simulink model "DCM_16_Series_Field_2"  (R2019b)
settings: Solver=VariableStepAuto  StartTime=0.0  StopTime=20  RelTol=1e-3
model workspace (MAT data in the model file):
  Laf = 0.00847
  Rarm = 0.0096
  angular_vel = 165
  angular_vel_13 = 163.55
  angular_vel_14 = 163.55
  angular_vel_15 = 163.55
  angular_vel_16 = 163.55
  angular_vel_2 = 165
libraries: powerlib x77, simulink x1
settings Model: Creator=Sy2  LastModifiedBy=Sy2
settings SolverCC: ZeroCrossAlgorithm=Adaptive
settings DebuggingCC: IgnoredZcDiagnostic=none

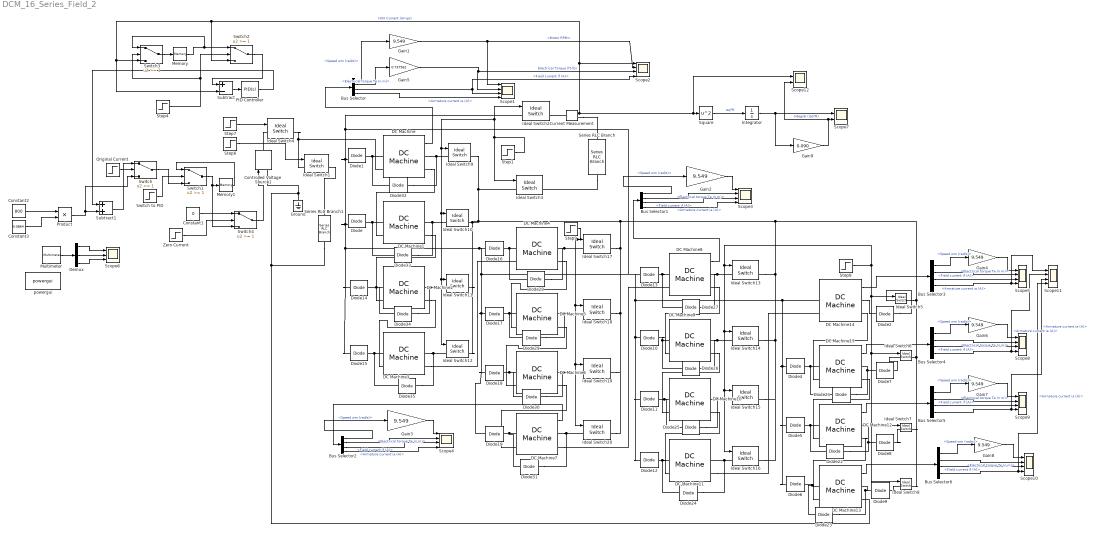
== system DCM_16_Series_Field_2 ==
  Bus Selector{,1..6} (7 alike) : BusSelector  OutputSignals=Speed wm (rad/s),Electrical torque Te (n m),Field current if (A),Armature current ia (A)
  Constant1 : Constant  Value=0
  Constant2 : Constant  Value=800
  Constant3 : Constant  Value=0.0864
  Controlled Voltage Source1 : powerlib/Electrical Sources/Controlled Voltage Source  Initialize=on  Source_Type=DC  Amplitude=0  Phase=0  Frequency=0  Measurements=Voltage
      settings: SourceProductName=Simscape Electrical
  Current Measurement : powerlib/Measurements/Current Measurement  PhasorSimulation=off  OutputType=Complex  PSBequivalent=0
      settings: SourceProductName=Simscape Electrical
  DC Machine{,1..13,15} (15 alike) : powerlib/Machines/DC Machine  PresetModel=No  MechanicalLoad=Torque TL  FieldType=Wound  ShowDetailedParameters=on  MeasurementBus=off  RLa="[Rarm  0.002]"  RLf=[0.0054 0.0125]  Laf=Laf  MachineConstant=Torque constant (N.m/A)  Ke=1.8  Kt=1.8  J=137  Bm=0  Tf=0  w0=angular_vel  Ifinit=0  TsPowergui=0  TsBlock=-1
      settings: SourceProductName=Simscape Electrical
  DC Machine14 : powerlib/Machines/DC Machine  PresetModel=No  MechanicalLoad=Torque TL  FieldType=Wound  ShowDetailedParameters=on  MeasurementBus=off  RLa="[Rarm  0.002]"  RLf=[0.0054 0.0125]  Laf=Laf  MachineConstant=Torque constant (N.m/A)  Ke=1.8  Kt=1.8  J=137  Bm=0  Tf=0  w0=angular_vel_13  Ifinit=0  TsPowergui=0  TsBlock=-1
      settings: SourceProductName=Simscape Electrical
  Demux : Demux  Outputs=3
  Diode : powerlib/Power Electronics/Diode  Ron=0.001  Lon=0  Vf=0.8  IC=0  UseSnubber=0  Rs=500  Cs=250e-9  Measurements=on
      settings: SourceProductName=Simscape Electrical
  Diode1 : powerlib/Power Electronics/Diode  Ron=0.001  Lon=0  Vf=0.8  IC=0  UseSnubber=0  Rs=500  Cs=250e-9  Measurements=on
      settings: SourceProductName=Simscape Electrical
  Diode{2,4..19,21..22} (19 alike) : powerlib/Power Electronics/Diode  Ron=0.001  Lon=0  Vf=0.8  IC=0  UseSnubber=0  Rs=500  Cs=250e-9  Measurements=off
      settings: SourceProductName=Simscape Electrical
  Diode{23..35} (13 alike) : powerlib/Power Electronics/Diode  Ron=0  Lon=0  Vf=0.8  IC=0  UseSnubber=0  Rs=500  Cs=250e-9  Measurements=off
      settings: SourceProductName=Simscape Electrical
  Gain{1..4,6..8} (7 alike) : Gain  Gain=9.549
  Gain5 : Gain  Gain=0.737562
  Gain9 : Gain  Gain=0.090
  Ground : powerlib/Elements/Ground  LConnTagsString=a
      settings: SourceProductName=Simscape Electrical
  Ideal Switch{1..3,5..20} (19 alike) : powerlib/Power Electronics/Ideal Switch  Ron=0  Lon=0  IC=0  Rs=inf  Cs=0  Measurements=on
      settings: SourceProductName=Simscape Electrical
  Ideal Switch4 : powerlib/Power Electronics/Ideal Switch  Ron=0  Lon=0  IC=1  Rs=inf  Cs=0  Measurements=on
      settings: SourceProductName=Simscape Electrical
  Integrator : Integrator  ZeroCross=off
  Memory : Memory
  Memory1 : Memory
  Multimeter : powerlib/Measurements/Multimeter  PhasorSimulation=off  OutputType=Complex  sel=[2 3 1]  L=3  Gain=[1 1 1]  yselected={'Usrc: Controlled Voltage Source1','Ib: Series RLC Branch1','Ub: Series RLC Branch1'};  PSBOutputType=1  PSBequivalent=0  AxesSetting=[0,0.1,-100,100]  Display=0  SavedBlockNames=-11
      settings: SourceProductName=Simscape Electrical
  Original Current : Step  Time=13  SampleTime=0  VectorParams1D=off  ZeroCross=off
  PID Controller : simulink/Continuous/PID Controller  Controller=PID  Form=Parallel  TimeDomain=Continuous-time  SampleTime=-1  IntegratorMethod=Forward Euler  FilterMethod=Forward Euler  ControllerParametersSource=internal  P=10  I=7  D=1  UseFilter=on  N=100  TunerSelectOption=Transfer Function Based (PID Tuner App)  InitialConditionSource=internal  InitialConditionForIntegrator=0  InitialConditionForFilter=0  DifferentiatorICPrevScaledInput=0  ExternalReset=none  TrackingMode=off  Kt=1  LimitOutput=off  UpperSaturationLimit=inf  LowerSaturationLimit=-inf  LinearizeAsGain=on  AntiWindupMode=none  Kb=1  POutMin=[]  POutMax=[]  IOutMin=[]  IOutMax=[]  DOutMin=[]  DOutMax=[]  NOutMin=[]  NOutMax=[]  SumOutMin=[]  SumOutMax=[]  SaturationOutMin=[]  SaturationOutMax=[]  PParamMin=[]  PParamMax=[]  IParamMin=[]  IParamMax=[]  DParamMin=[]  DParamMax=[]  NParamMin=[]  NParamMax=[]  KbParamMin=[]  KbParamMax=[]  KtParamMin=[]  KtParamMax=[]  KbOutMin=[]  KbOutMax=[]  KtOutMin=[]  KtOutMax=[]  IntegratorOutMin=[]  IntegratorOutMax=[]  FilterOutMin=[]  FilterOutMax=[]  SumI1OutMin=[]  SumI1OutMax=[]  SumI2OutMin=[]  SumI2OutMax=[]  SumI3OutMin=[]  SumI3OutMax=[]  SumI4OutMin=[]  SumI4OutMax=[]  SumDOutMin=[]  SumDOutMax=[]  DifferentiatorOutMin=[]  DifferentiatorOutMax=[]  FilterDiffOutCoefMin=[]  FilterDiffOutCoefMax=[]  ReciprocalOutMin=[]  ReciprocalOutMax=[]  SumDenOutMin=[]  SumDenOutMax=[]  SumNumOutMin=[]  SumNumOutMax=[]  DivideOutMin=[]  DivideOutMax=[]  IntegratorContinuousStateAttributes=''  IntegratorStateMustResolveToSignalObject=off  IntegratorRTWStateStorageClass=Auto  FilterContinuousStateAttributes=''  FilterStateMustResolveToSignalObject=off  FilterRTWStateStorageClass=Auto  ParallelPVariant=InternalParameters  IdealPVariant=Disabled  IVariant=InternalParameters  DVariant=InternalParameters  IntegratorVariant=Continuous  SatVariant=Disabled  AWVariant=Passthrough  PCopyVariant=Disabled  TRVariant=Disabled  FdbkBlocksVariant=Forward  IdealPFdbkVariant=Disabled  SatFdbkVariant=Disabled  DerivativeFilterVariant=ContFilter  NVariant=InternalParameters  NCopyVariant=Disabled  FilterICVariant=InternalICsFilter  IntegratorICVariant=InternalICs  ExternalResetVariant=Disabled  TRSumVariant=Passthrough  SumFdbkVariant=Disabled  SumVariant=Sum_PID
  Product : Product
  Scope{1..5,8..11} (9 alike) : Scope  NumInputPorts=4
  Scope12 : Scope  NumInputPorts=2
  Scope6 : Scope  NumInputPorts=3
  Scope7 : Scope  NumInputPorts=2
  Series RLC Branch : powerlib/Elements/Series RLC Branch  LConnTagsString=__new0  RConnTagsString=__new0  BranchType=RL  Resistance=0.09  Inductance=0.02  SetiL0=off  InitialCurrent=0  Capacitance=1e-6  Setx0=off  InitialVoltage=0  Measurements=None
      settings: SourceProductName=Simscape Electrical
  Series RLC Branch1 : powerlib/Elements/Series RLC Branch  Description=Field Dump Resistor  LConnTagsString=__new0  RConnTagsString=__new0  BranchType=R  Resistance=5  Inductance=1e-3  SetiL0=off  InitialCurrent=0  Capacitance=1e-6  Setx0=off  InitialVoltage=0  Measurements=Branch voltage and current
      settings: AttributesFormatString=%<Description>  SourceProductName=Simscape Electrical
  Square : Math  Operator=square  RndMeth=Zero  SaturateOnIntegerOverflow=on
  Step1 : Step  Time=12  SampleTime=0  VectorParams1D=off
  Step4 : Step  Time=12.72  SampleTime=0  VectorParams1D=off  ZeroCross=off
  Step6 : Step  Time=12.85  SampleTime=0  VectorParams1D=off  ZeroCross=off
  Step7 : Step  Time=13  Before=1  After=0  SampleTime=0  VectorParams1D=off  ZeroCross=off
  Step8 : Step  Time=12  SampleTime=0  VectorParams1D=off
  Step9 : Step  Time=12  SampleTime=0  VectorParams1D=off
  Subtract : Sum  Inputs=+-
  Subtract1 : Sum
  Switch{,1..4} (5 alike) : Switch  Threshold=1  ZeroCross=off
  Switch to PID : Step  Time=13  SampleTime=0  VectorParams1D=off  ZeroCross=off
  Zero Current : Step  Time=13  SampleTime=0  VectorParams1D=off  ZeroCross=off
  powergui : powerlib/powergui  Priority=1  SimulationMode=Continuous  SampleTime=50e-6  frequency=60  Iterations=50  frequencyindice=0  Pbase=100e6  ErrMax=1e-4  UnitsV=kV  UnitsW=MW  buscounter=0  FunctionMessages=off  echomessages=off  EnableUseOfTLC=off  CurrentSourceSwitches=off  DisableSnubberDevices=off  DisableRonSwitches=off  DisableVfSwitches=off  DisplayEquations=off  AutomaticDiscreteSolvers=off  SolverType=Tustin/Backward Euler (TBE)  Interpol=off  ExternalGateDelay=off  methode=off  Ts=100  x0status=blocks  SPID=on  SwTol=0  HookPort=off  NonlinearTolerance=1e-4  nMaxIteration=100  ContinueOnMaxIteration=off  RestoreLinks=warning  ResistiveCurrentMeasurement=off  Frange=[0:2:500]  Ylog=off  Xlog=on  ShowGrid=off  save=off  variable=ZData  structure=0  ZoomFFT=off  StartTime=0.0  cycles=1  DisplayStyle=1  fundamental=60  FreqAxis=off  MaxFrequency=1000  frequencyindicesteady=1  RmsSteady=1  display=off
      settings: SourceProductName=Simscape Electrical
  wires:
  DC Machine/1 -> Bus Selector/1
  Bus Selector/1 -> Gain1/1  "<Speed wm (rad/s)>"
  Bus Selector/3 -> Scope2/4, Scope1/3  "<Field current if (A)>"
  Bus Selector/4 -> Scope1/4  "<Armature current ia (A)>"
  Gain1/1 -> Scope1/1, Scope2/2  "<Motor RPM>"
  Step1/1 -> Ideal Switch10/1, Ideal Switch11/1, Ideal Switch12/1, Ideal Switch9/1, Ideal Switch2/1, Ideal Switch3/1
  Original Current/1 -> Switch/2
  Current Measurement/1 -> Scope12/1, Square/1, Switch2/3, Switch3/3, Subtract/2, Scope2/1  "HSX Current (Amps)"
  DC Machine8/1 -> Bus Selector1/1
  Bus Selector1/4 -> Scope3/4  "<Armature current ia (A)>"
  Bus Selector1/1 -> Gain2/1  "<Speed wm (rad/s)>"
  Bus Selector1/2 -> Scope3/2  "<Electrical torque Te (n m)>"
  Gain2/1 -> Scope3/1
  Bus Selector1/3 -> Scope3/3  "<Field current if (A)>"
  Bus Selector2/4 -> Scope4/4  "<Armature current ia (A)>"
  Bus Selector2/2 -> Scope4/2  "<Electrical torque Te (n m)>"
  Gain3/1 -> Scope4/1
  Bus Selector2/3 -> Scope4/3  "<Field current if (A)>"
  DC Machine7/1 -> Bus Selector2/1
  Bus Selector2/1 -> Gain3/1  "<Speed wm (rad/s)>"
  Memory/1 -> Switch3/1, Switch2/1
  Subtract/1 -> PID Controller/1
  PID Controller/1 -> Subtract1/1
  Constant2/1 -> Product/1
  Subtract1/1 -> Switch/1
  Switch to PID/1 -> Switch1/2
  Switch2/1 -> Subtract/1
  Step4/1 -> Switch2/2, Switch3/2
  Switch3/1 -> Memory/1
  Bus Selector/2 -> Gain5/1  "<Electrical torque Te (n m)>"
  Gain5/1 -> Scope1/2, Scope2/3  "Electrical Torque (ft-lb)"
  Square/1 -> Integrator/1  "Isq*R"
  Switch4/1 -> Controlled Voltage Source1/1
  Zero Current/1 -> Switch4/2
  Constant1/1 -> Switch4/1
  Step6/1 -> Ideal Switch1/1
  Step7/1 -> Ideal Switch4/1
  Constant3/1 -> Product/2
  Product/1 -> Subtract1/2, Switch/3
  Switch/1 -> Switch1/3
  Switch1/1 -> Switch4/3, Memory1/1
  Memory1/1 -> Switch1/1
  Demux/2 -> Scope6/2
  Multimeter/1 -> Demux/1
  Demux/1 -> Scope6/1
  Demux/3 -> Scope6/3
  Gain6/1 -> Scope8/1
  DC Machine15/1 -> Bus Selector4/1
  Bus Selector4/4 -> Scope11/2, Scope8/4  "<Armature current ia (A)>"
  Bus Selector4/1 -> Gain6/1  "<Speed wm (rad/s)>"
  Bus Selector4/2 -> Scope8/2  "<Electrical torque Te (n m)>"
  Bus Selector4/3 -> Scope8/3  "<Field current if (A)>"
  Bus Selector5/3 -> Scope9/3  "<Field current if (A)>"
  DC Machine12/1 -> Bus Selector5/1
  Gain7/1 -> Scope9/1
  Bus Selector5/2 -> Scope9/2  "<Electrical torque Te (n m)>"
  Bus Selector5/1 -> Gain7/1  "<Speed wm (rad/s)>"
  Bus Selector5/4 -> Scope11/3, Scope9/4  "<Armature current ia (A)>"
  Bus Selector6/4 -> Scope11/4, Scope10/4  "<Armature current ia (A)>"
  Gain8/1 -> Scope10/1
  Bus Selector6/1 -> Gain8/1  "<Speed wm (rad/s)>"
  Bus Selector6/2 -> Scope10/2  "<Electrical torque Te (n m)>"
  Bus Selector6/3 -> Scope10/3  "<Field current if (A)>"
  DC Machine13/1 -> Bus Selector6/1
  Bus Selector3/3 -> Scope5/3  "<Field current if (A)>"
  DC Machine14/1 -> Bus Selector3/1
  Gain4/1 -> Scope5/1
  Bus Selector3/2 -> Scope5/2  "<Electrical torque Te (n m)>"
  Bus Selector3/1 -> Gain4/1  "<Speed wm (rad/s)>"
  Bus Selector3/4 -> Scope11/1, Scope5/4  "<Armature current ia (A)>"
  Step8/1 -> Ideal Switch14/1, Ideal Switch15/1, Ideal Switch16/1, Ideal Switch13/1, Ideal Switch8/1, Ideal Switch7/1, Ideal Switch6/1, Ideal Switch5/1
  Step9/1 -> Ideal Switch19/1, Ideal Switch20/1, Ideal Switch18/1, Ideal Switch17/1
  Integrator/1 -> Gain9/1, Scope7/1
  Gain9/1 -> Scope12/2, Scope7/2  "Integral (Isq*R)"
  connections:
  Ideal Switch3/LConn1 -- Ideal Switch9/RConn1 -- Ideal Switch17/RConn1 -- Ideal Switch18/RConn1 -- Ideal Switch19/RConn1 -- Ideal Switch20/RConn1 -- Ideal Switch8/RConn1 -- Ideal Switch7/RConn1 -- Ideal Switch6/RConn1 -- Ideal Switch5/RConn1 -- Ideal Switch13/RConn1 -- Ideal Switch14/RConn1 -- Ideal Switch15/RConn1 -- Ideal Switch16/RConn1 -- Ideal Switch12/RConn1 -- Ideal Switch11/RConn1 -- Ideal Switch10/RConn1
  Series RLC Branch/RConn1 -- Ideal Switch3/RConn1
  Current Measurement/LConn1 -- Ideal Switch2/RConn1
  Current Measurement/RConn1 -- Series RLC Branch/LConn1
  DC Machine/RConn2 -- DC Machine1/LConn2
  DC Machine1/RConn2 -- DC Machine2/LConn2
  DC Machine2/RConn2 -- DC Machine3/LConn2
  DC Machine3/RConn2 -- DC Machine4/LConn2
  DC Machine4/RConn2 -- DC Machine5/LConn2
  DC Machine5/RConn2 -- DC Machine6/LConn2
  DC Machine6/RConn2 -- DC Machine7/LConn2
  DC Machine7/RConn2 -- DC Machine8/LConn2
  DC Machine8/RConn2 -- DC Machine9/LConn2
  DC Machine9/RConn2 -- DC Machine10/LConn2
  DC Machine10/RConn2 -- DC Machine11/LConn2
  DC Machine11/RConn2 -- DC Machine14/LConn2
  DC Machine14/RConn2 -- DC Machine15/LConn2
  DC Machine15/RConn2 -- DC Machine12/LConn2
  DC Machine12/RConn2 -- DC Machine13/LConn2
  DC Machine/LConn2 -- Ideal Switch4/RConn1 -- Ideal Switch1/LConn1
  Ground/LConn1 -- Series RLC Branch1/RConn1 -- DC Machine13/RConn2 -- Controlled Voltage Source1/LConn1
  Ideal Switch1/RConn1 -- Series RLC Branch1/LConn1
  Controlled Voltage Source1/RConn1 -- Ideal Switch4/LConn1
  Ideal Switch9/LConn1 -- Diode32/LConn1 -- DC Machine/RConn1
  Ideal Switch10/LConn1 -- Diode33/LConn1 -- DC Machine1/RConn1
  Ideal Switch11/LConn1 -- Diode34/LConn1 -- DC Machine2/RConn1
  DC Machine3/RConn1 -- Diode35/LConn1 -- Ideal Switch12/LConn1
  Ideal Switch13/LConn1 -- Diode27/LConn1 -- DC Machine8/RConn1
  Ideal Switch14/LConn1 -- Diode26/LConn1 -- DC Machine9/RConn1
  Ideal Switch15/LConn1 -- Diode25/LConn1 -- DC Machine10/RConn1
  Ideal Switch16/LConn1 -- Diode24/LConn1 -- DC Machine11/RConn1
  DC Machine7/RConn1 -- Diode31/LConn1 -- Ideal Switch20/LConn1
  DC Machine6/RConn1 -- Ideal Switch19/LConn1 -- Diode30/LConn1
  DC Machine5/RConn1 -- Ideal Switch18/LConn1 -- Diode29/LConn1
  DC Machine4/RConn1 -- Ideal Switch17/LConn1 -- Diode28/LConn1
  Diode/LConn1 -- Diode33/RConn1 -- DC Machine1/LConn1
  Diode1/LConn1 -- Diode32/RConn1 -- DC Machine/LConn1
  Diode4/LConn1 -- Diode21/RConn1 -- DC Machine15/LConn1
  Diode5/LConn1 -- Diode22/RConn1 -- DC Machine12/LConn1
  DC Machine13/LConn1 -- Diode6/LConn1 -- Diode23/RConn1
  Diode7/RConn1 -- Diode21/LConn1 -- DC Machine15/RConn1
  Ideal Switch6/LConn1 -- Diode7/LConn1
  Diode8/LConn1 -- Ideal Switch7/LConn1
  Diode8/RConn1 -- Diode22/LConn1 -- DC Machine12/RConn1
  Diode9/LConn1 -- Ideal Switch8/LConn1
  Diode9/RConn1 -- DC Machine13/RConn1 -- Diode23/LConn1
  Diode10/LConn1 -- Diode26/RConn1 -- DC Machine9/LConn1
  Diode11/LConn1 -- DC Machine10/LConn1 -- Diode25/RConn1
  Diode12/LConn1 -- Diode24/RConn1 -- DC Machine11/LConn1
  Diode13/LConn1 -- Diode27/RConn1 -- DC Machine8/LConn1
  DC Machine2/LConn1 -- Diode14/LConn1 -- Diode34/RConn1
  DC Machine3/LConn1 -- Diode35/RConn1 -- Diode15/LConn1
  Diode16/LConn1 -- Diode28/RConn1 -- DC Machine4/LConn1
  Diode17/LConn1 -- Diode29/RConn1 -- DC Machine5/LConn1
  Diode18/LConn1 -- Diode30/RConn1 -- DC Machine6/LConn1
  DC Machine7/LConn1 -- Diode31/RConn1 -- Diode19/LConn1
  DC Machine14/LConn1 -- Diode6/RConn1 -- Diode5/RConn1 -- Diode4/RConn1 -- Diode12/RConn1 -- Diode11/RConn1 -- Diode10/RConn1 -- Diode17/RConn1 -- Diode18/RConn1 -- Diode19/RConn1 -- Diode16/RConn1 -- Diode14/RConn1 -- Diode15/RConn1 -- Diode/RConn1 -- Diode1/RConn1 -- Ideal Switch2/LConn1 -- Diode13/RConn1
  DC Machine14/RConn1 -- Diode2/RConn1
  Diode2/LConn1 -- Ideal Switch5/LConn1
